simulink model "Schema_Complet3"  (R2016b)
settings: Solver=VariableStepAuto  StartTime=0.0  StopTime=0.2  MaxStep=1e-4  RelTol=1e-3  EnableMultiTasking=on
values from neighbouring files (symbols this model uses):
  K1 = 856    [bode_param.m]    (also in reponse_temp.m)
  Kp2 = 10^(-1.5)    (= 0.0316227766017)    [bode_param.m]
  Ti = 1    [bode_param.m]    (also in reponse_temp.m)
  Tm = 3*1E-2    (= 0.03)    [bode_param.m]    (also in reponse_temp.m)
  Zc0 = 0.050    (= 0.05)    [bode_param.m]    (also in reponse_temp.m)
libraries: simulink x1
settings Model: Creator=pt_ptsi  LastModifiedBy=emiliendurif
settings DataIOCC: LimitDataPoints=on
settings OptimizationCC: LifeSpan=inf
settings DebuggingCC: AllowSymbolicDim=off  SFUnexpectedBacktrackingDiag=warning  SFNoUnconditionalDefaultTransitionDiag=warning  SFExecutionAtInitializationDiag=none
settings ModelReferenceCC: PropagateSignalLabelsOutOfModel=off
settings GRTTargetCC: TargetLangStandard=C89/C90 (ANSI)
settings ConfigComp: CovMetricSettings=dw  CovHtmlReporting=on  CovSaveCumulativeToWorkspaceVar=on  CovSaveSingleToWorkspaceVar=on  CovExternalEMLEnable=off

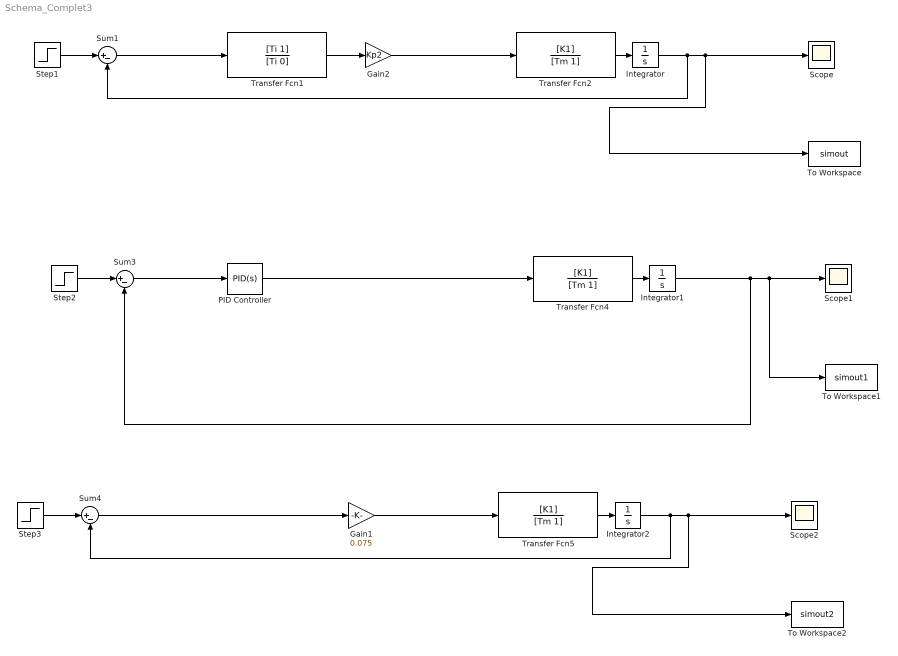
== system Schema_Complet3 ==
  Gain1 : Gain  Gain=0.075
  Gain2 : Gain  Gain=Kp2
  Integrator : Integrator
  Integrator1 : Integrator
  Integrator2 : Integrator
  PID Controller : simulink/Continuous/PID Controller  Controller=PID  TimeDomain=Continuous-time  SampleTime=-1  IntegratorMethod=Forward Euler  FilterMethod=Forward Euler  Form=Parallel  UseFilter=on  ControllerParametersSource=internal  P=0.189080626075099  I=2.11144406419596  D=0.00379920180701313  N=1186.61590095346  InitialConditionSource=internal  InitialConditionForIntegrator=0  InitialConditionForFilter=0  ExternalReset=none  LimitOutput=off  UpperSaturationLimit=inf  LowerSaturationLimit=-inf  LinearizeAsGain=on  AntiWindupMode=none  Kb=1  TrackingMode=off  Kt=1  PParamMin=[]  PParamMax=[]  IParamMin=[]  IParamMax=[]  DParamMin=[]  DParamMax=[]  NParamMin=[]  NParamMax=[]  KbParamMin=[]  KbParamMax=[]  KtParamMin=[]  KtParamMax=[]  POutMin=[]  POutMax=[]  IOutMin=[]  IOutMax=[]  DOutMin=[]  DOutMax=[]  NOutMin=[]  NOutMax=[]  KbOutMin=[]  KbOutMax=[]  KtOutMin=[]  KtOutMax=[]  IntegratorOutMin=[]  IntegratorOutMax=[]  FilterOutMin=[]  FilterOutMax=[]  SumOutMin=[]  SumOutMax=[]  SumI1OutMin=[]  SumI1OutMax=[]  SumI2OutMin=[]  SumI2OutMax=[]  SumI3OutMin=[]  SumI3OutMax=[]  SumDOutMin=[]  SumDOutMax=[]  SaturationOutMin=[]  SaturationOutMax=[]  IntegratorContinuousStateAttributes=''  IntegratorStateMustResolveToSignalObject=off  IntegratorRTWStateStorageClass=Auto  FilterContinuousStateAttributes=''  FilterStateMustResolveToSignalObject=off  FilterRTWStateStorageClass=Auto  DifferentiatorICPrevScaledInput=0  DifferentiatorOutMin=[]  DifferentiatorOutMax=[]
  Scope : Scope
  Scope1 : Scope
  Scope2 : Scope
  Step1 : Step  Time=0  After=Zc0  SampleTime=0
  Step2 : Step  Time=0  After=Zc0  SampleTime=0
  Step3 : Step  Time=0  After=Zc0  SampleTime=0
  Sum1 : Sum  Inputs=|+-
  Sum3 : Sum  Inputs=|+-
  Sum4 : Sum  Inputs=|+-
  To Workspace : ToWorkspace  VariableName=simout  SaveFormat=Timeseries  SampleTime=-1
  To Workspace1 : ToWorkspace  VariableName=simout1  SaveFormat=Timeseries  SampleTime=-1
  To Workspace2 : ToWorkspace  VariableName=simout2  SaveFormat=Timeseries  SampleTime=-1
  Transfer Fcn1 : TransferFcn  Numerator=[Ti 1]  Denominator=[Ti 0]
  Transfer Fcn2 : TransferFcn  Numerator=[K1]  Denominator=[Tm 1]
  Transfer Fcn4 : TransferFcn  Numerator=[K1]  Denominator=[Tm 1]
  Transfer Fcn5 : TransferFcn  Numerator=[K1]  Denominator=[Tm 1]
  wires:
  Transfer Fcn1/1 -> Gain2/1
  Step1/1 -> Sum1/1
  Gain2/1 -> Transfer Fcn2/1
  Sum1/1 -> Transfer Fcn1/1
  Transfer Fcn2/1 -> Integrator/1
  Integrator/1 -> Sum1/2, To Workspace/1, Scope/1
  Step2/1 -> Sum3/1
  PID Controller/1 -> Transfer Fcn4/1
  Transfer Fcn4/1 -> Integrator1/1
  Integrator1/1 -> Sum3/2, To Workspace1/1, Scope1/1
  Sum3/1 -> PID Controller/1
  Sum4/1 -> Gain1/1
  Step3/1 -> Sum4/1
  Gain1/1 -> Transfer Fcn5/1
  Transfer Fcn5/1 -> Integrator2/1
  Integrator2/1 -> Sum4/2, To Workspace2/1, Scope2/1
